simulink model "to_line_segments"  (R2018a)
settings: Solver=VariableStepAuto  StartTime=0.0  StopTime=120  FixedStep=0.01  MaxStep=.01  RelTol=1e-3
settings Model: Creator=U500304  LastModifiedBy=U500304
settings SolverCC: ZeroCrossAlgorithm=Adaptive
settings DataIOCC: SaveOutput=off  SaveTime=off
settings DebuggingCC: MaxConsecutiveZCsMsg=warning

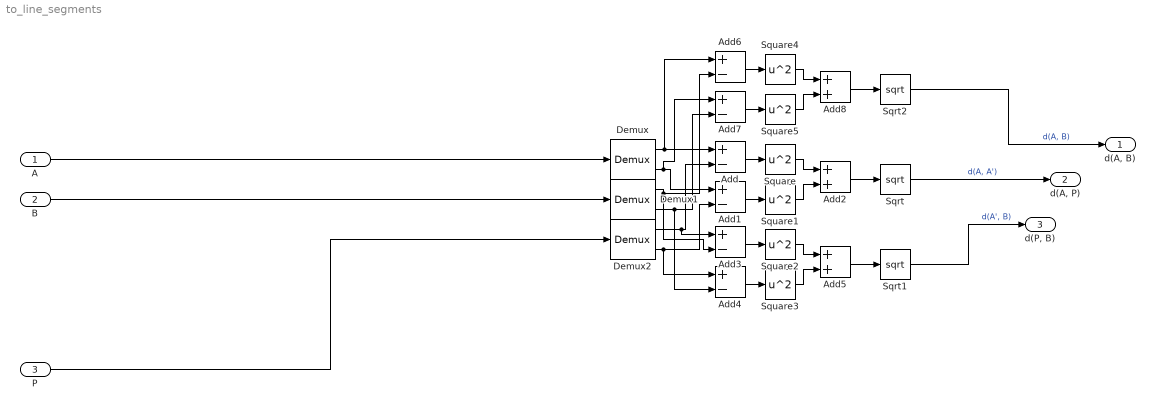
== system to_line_segments ==
  A : Inport  OutDataTypeStr=double  PortDimensions=2
  B : Inport  Port=2  OutDataTypeStr=double  PortDimensions=2
  P : Inport  Port=3  OutDataTypeStr=double  PortDimensions=2
  Add{,1,3..4,6..7} (6 alike) : Sum  Inputs=+-
  Add2 : Sum
  Add5 : Sum
  Add8 : Sum
  Demux : Demux  Outputs=2
  Demux1 : Demux  Outputs=2
  Demux2 : Demux  Outputs=2
  Sqrt : Sqrt  SaturateOnIntegerOverflow=on
  Sqrt1 : Sqrt  SaturateOnIntegerOverflow=on
  Sqrt2 : Sqrt  SaturateOnIntegerOverflow=on
  Square{,1..5} (6 alike) : Math  Operator=square  SaturateOnIntegerOverflow=on
  "d(A, B)" : Outport  OutDataTypeStr=double  PortDimensions=1
  "d(A, P)" : Outport  Port=2  OutDataTypeStr=double  PortDimensions=1
  "d(P, B)" : Outport  Port=3  OutDataTypeStr=double  PortDimensions=1
  wires:
  Sqrt/1 -> "d(A, P)"/1  "d(A, A')"
  Demux/2 -> Add1/1, Add7/1
  B/1 -> Demux1/1
  Square/1 -> Add2/1
  Add2/1 -> Sqrt/1
  Demux/1 -> Add/1, Add6/1
  P/1 -> Demux2/1
  Add3/1 -> Square2/1
  Add8/1 -> Sqrt2/1
  Sqrt1/1 -> "d(P, B)"/1  "d(A', B)"
  Demux2/2 -> Add1/2, Add4/1
  Demux2/1 -> Add/2, Add3/1
  Add/1 -> Square/1
  Add1/1 -> Square1/1
  Square1/1 -> Add2/2
  Demux1/1 -> Add3/2, Add6/2
  A/1 -> Demux/1
  Square3/1 -> Add5/2
  Add5/1 -> Sqrt1/1
  Square2/1 -> Add5/1
  Add6/1 -> Square4/1
  Square5/1 -> Add8/2
  Add4/1 -> Square3/1
  Demux1/2 -> Add4/2, Add7/2
  Square4/1 -> Add8/1
  Add7/1 -> Square5/1
  Sqrt2/1 -> "d(A, B)"/1  "d(A, B)"
